simulink model "bilat_teleop_time_delay"  (R2017a)
settings: Solver=VariableStepAuto  StartTime=0.0  StopTime=100  MaxStep=0.05  RelTol=1e-3
values from neighbouring files (symbols this model uses):
  Bm = [1 0; 0 1]    [bilat_teleop_multiDOF_params.m]    (also in bilat_teleop_time_delay_params.m = 0; sampled_data_bilat_teleop_tavakoli_params.m = 0.1; sampled_data_bilat_teleop_time_delay_params.m = 0.1)
  Bs = [1 0; 0 1]    [bilat_teleop_multiDOF_params.m]    (also in bilat_teleop_time_delay_params.m = 0; sampled_data_bilat_teleop_tavakoli_params.m = 0.1; sampled_data_bilat_teleop_time_delay_params.m = 0.1)
  Km = 0    [bilat_teleop_time_delay_params.m]
  Ks = 0    [bilat_teleop_time_delay_params.m]
  Mm = 1    [bilat_teleop_time_delay_params.m]    (also in sampled_data_bilat_teleop_tavakoli_params.m = 0.015; sampled_data_bilat_teleop_time_delay_params.m = 0.015)
  Ms = 1    [bilat_teleop_time_delay_params.m]    (also in sampled_data_bilat_teleop_tavakoli_params.m = 0.015; sampled_data_bilat_teleop_time_delay_params.m = 0.015)
libraries: simulink x1
settings Model: Creator=salou  LastModifiedBy=salou

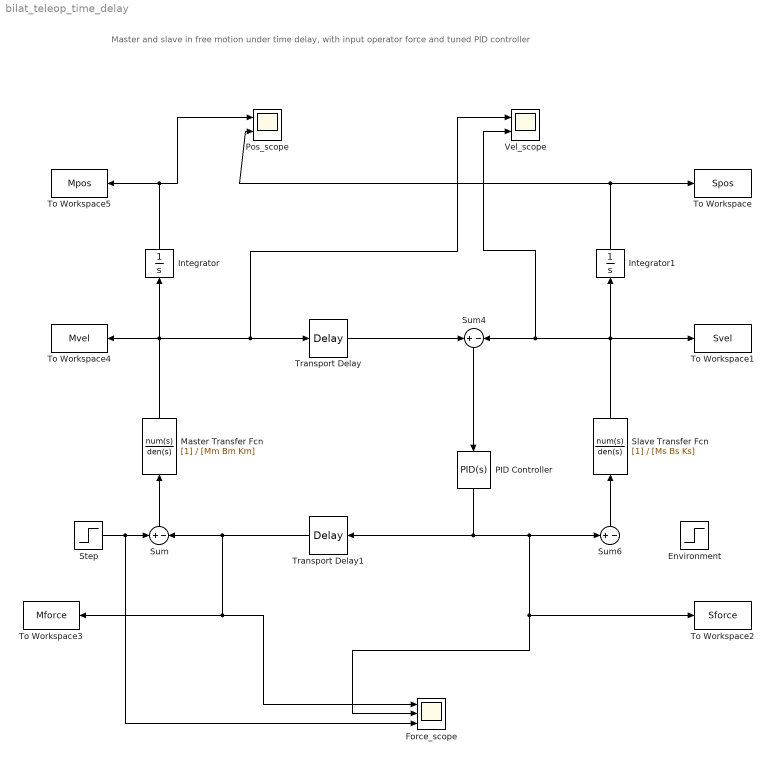
== system bilat_teleop_time_delay ==
  note: Master and slave in free motion under time delay, with input operator force and tuned PID controller
  Environment : Step  SampleTime=0
  Force_scope : Scope  NumInputPorts=3
  Integrator : Integrator
  Integrator1 : Integrator
  Master Transfer Fcn : TransferFcn  Denominator=[Mm Bm Km]
  PID Controller : simulink/Continuous/PID Controller  Controller=PID  TimeDomain=Continuous-time  SampleTime=-1  IntegratorMethod=Forward Euler  FilterMethod=Forward Euler  Form=Parallel  UseFilter=on  ControllerParametersSource=internal  P=1.044  I=0.1213  D=1.56681262957778  N=3.24752514262653  InitialConditionSource=internal  InitialConditionForIntegrator=0  InitialConditionForFilter=0  ExternalReset=none  LimitOutput=off  UpperSaturationLimit=inf  LowerSaturationLimit=-inf  LinearizeAsGain=on  AntiWindupMode=none  Kb=1  TrackingMode=off  Kt=1  PParamMin=[]  PParamMax=[]  IParamMin=[]  IParamMax=[]  DParamMin=[]  DParamMax=[]  NParamMin=[]  NParamMax=[]  KbParamMin=[]  KbParamMax=[]  KtParamMin=[]  KtParamMax=[]  POutMin=[]  POutMax=[]  IOutMin=[]  IOutMax=[]  DOutMin=[]  DOutMax=[]  NOutMin=[]  NOutMax=[]  KbOutMin=[]  KbOutMax=[]  KtOutMin=[]  KtOutMax=[]  IntegratorOutMin=[]  IntegratorOutMax=[]  FilterOutMin=[]  FilterOutMax=[]  SumOutMin=[]  SumOutMax=[]  SumI1OutMin=[]  SumI1OutMax=[]  SumI2OutMin=[]  SumI2OutMax=[]  SumI3OutMin=[]  SumI3OutMax=[]  SumDOutMin=[]  SumDOutMax=[]  SaturationOutMin=[]  SaturationOutMax=[]  IntegratorContinuousStateAttributes=''  IntegratorStateMustResolveToSignalObject=off  IntegratorRTWStateStorageClass=Auto  FilterContinuousStateAttributes=''  FilterStateMustResolveToSignalObject=off  FilterRTWStateStorageClass=Auto  DifferentiatorICPrevScaledInput=0  DifferentiatorOutMin=[]  DifferentiatorOutMax=[]  InitialConditionSetting=State (most efficient)
  Pos_scope : Scope  NumInputPorts=2
  Slave Transfer Fcn : TransferFcn  Denominator=[Ms Bs Ks]
  Step : Step  SampleTime=0
  Sum : Sum  Inputs=+|-
  Sum4 : Sum  Inputs=+|-
  Sum6 : Sum  Inputs=+|-
  To Workspace : ToWorkspace  VariableName=Spos  SaveFormat=Timeseries  SampleTime=-1
  To Workspace1 : ToWorkspace  VariableName=Svel  SaveFormat=Timeseries  SampleTime=-1
  To Workspace2 : ToWorkspace  VariableName=Sforce  SaveFormat=Timeseries  SampleTime=-1
  To Workspace3 : ToWorkspace  VariableName=Mforce  SaveFormat=Timeseries  SampleTime=-1
  To Workspace4 : ToWorkspace  VariableName=Mvel  SaveFormat=Timeseries  SampleTime=-1
  To Workspace5 : ToWorkspace  VariableName=Mpos  SaveFormat=Timeseries  SampleTime=-1
  Transport Delay : TransportDelay  DelayTime=5
  Transport Delay1 : TransportDelay  DelayTime=5
  Vel_scope : Scope  NumInputPorts=2
  wires:
  Step/1 -> Force_scope/3, Sum/1
  ? -> Sum6/2
  Transport Delay1/1 -> Force_scope/1, To Workspace3/1, Sum/2
  Sum/1 -> Master Transfer Fcn/1
  Master Transfer Fcn/1 -> To Workspace4/1, Vel_scope/1, Transport Delay/1, Integrator/1
  Transport Delay/1 -> Sum4/1
  PID Controller/1 -> Transport Delay1/1, To Workspace2/1, Force_scope/2, Sum6/1
  Sum6/1 -> Slave Transfer Fcn/1
  Slave Transfer Fcn/1 -> To Workspace1/1, Integrator1/1, Sum4/2, Vel_scope/2
  Integrator/1 -> Pos_scope/1, To Workspace5/1
  Integrator1/1 -> To Workspace/1, Pos_scope/2
  Sum4/1 -> PID Controller/1
